simulink model "m20192020"  (R2016a)
settings: Solver=FixedStepAuto  StartTime=0.0  StopTime=0.5  FixedStep=0.01  RelTol=1e-3
settings Model: Creator=witkey721  LastModifiedBy=witkey721

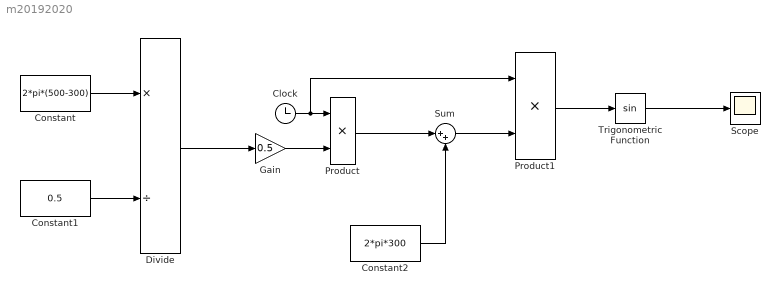
== system m20192020 ==
  Clock : Clock
  Constant : Constant  Value=2*pi*(500-300)
  Constant1 : Constant  Value=0.5
  Constant2 : Constant  Value=2*pi*300
  Divide : Product  Inputs=*/
  Gain : Gain  Gain=0.5
  Product : Product
  Product1 : Product
  Scope : Scope
  Sum : Sum  Inputs=|++
  Trigonometric Function : Trigonometry
  wires:
  Constant/1 -> Divide/1
  Constant1/1 -> Divide/2
  Divide/1 -> Gain/1
  Gain/1 -> Product/2
  Clock/1 -> Product1/1, Product/1
  Product/1 -> Sum/1
  Constant2/1 -> Sum/2
  Sum/1 -> Product1/2
  Product1/1 -> Trigonometric Function/1
  Trigonometric Function/1 -> Scope/1
